simulink model "lookup_nD_TestGen39"  (R2017b)
settings: Solver=FixedStepDiscrete  StartTime=0.0  StopTime=10.0  RelTol=1e-3
model workspace (MAT data in the model file):
  LUTObjLKnD39 = Simulink.LookupTable
  LUTObjLKnD39.Table = Simulink.lookuptable.Table
  LUTObjLKnD39.Table.Value = [4 16 10 4 16 10 4 16 10 4 16 10 ... (2160 elements, 2x5x3x2x3x4x3)]
  LUTObjLKnD39.Table.Dimensions = [2 5 3 2 3 4 3]
  LUTObjLKnD39.Table.DataType = 'double'
  LUTObjLKnD39.Table.FieldName = 'Table'
  LUTObjLKnD39.Breakpoints(1) = Simulink.lookuptable.Breakpoint
  LUTObjLKnD39.Breakpoints(1).Value = [61.721962121; 104.300096243]
  LUTObjLKnD39.Breakpoints(1).TunableSizeName = 'N1'
  LUTObjLKnD39.Breakpoints(1).Dimensions = [2 1]
  LUTObjLKnD39.Breakpoints(1).DataType = 'double'
  LUTObjLKnD39.Breakpoints(1).FieldName = 'BP1'
  LUTObjLKnD39.Breakpoints(2) = Simulink.lookuptable.Breakpoint
  LUTObjLKnD39.Breakpoints(2).Value = [37.260919995; 59.6796023238; 63.5646368852; 96.2573922912; 103.388327939]
  LUTObjLKnD39.Breakpoints(2).TunableSizeName = 'N2'
  LUTObjLKnD39.Breakpoints(2).Dimensions = [5 1]
  LUTObjLKnD39.Breakpoints(2).DataType = 'double'
  LUTObjLKnD39.Breakpoints(2).FieldName = 'BP2'
  LUTObjLKnD39.Breakpoints(3) = Simulink.lookuptable.Breakpoint
  LUTObjLKnD39.Breakpoints(3).Value = [0.658816623389; 20.0277443068; 89.2681267122]
  LUTObjLKnD39.Breakpoints(3).TunableSizeName = 'N3'
  LUTObjLKnD39.Breakpoints(3).Dimensions = [3 1]
  LUTObjLKnD39.Breakpoints(3).DataType = 'double'
  LUTObjLKnD39.Breakpoints(3).FieldName = 'BP3'
  LUTObjLKnD39.Breakpoints(4) = Simulink.lookuptable.Breakpoint
  LUTObjLKnD39.Breakpoints(4).Value = [83.69732351; 108.985900351]
  LUTObjLKnD39.Breakpoints(4).TunableSizeName = 'N4'
  LUTObjLKnD39.Breakpoints(4).Dimensions = [2 1]
  LUTObjLKnD39.Breakpoints(4).DataType = 'double'
  LUTObjLKnD39.Breakpoints(4).FieldName = 'BP4'
  LUTObjLKnD39.Breakpoints(5) = Simulink.lookuptable.Breakpoint
  LUTObjLKnD39.Breakpoints(5).Value = [49.9740707452; 87.8847504391; 124.596963914]
  LUTObjLKnD39.Breakpoints(5).TunableSizeName = 'N5'
  LUTObjLKnD39.Breakpoints(5).Dimensions = [3 1]
  LUTObjLKnD39.Breakpoints(5).DataType = 'double'
  LUTObjLKnD39.Breakpoints(5).FieldName = 'BP5'
  LUTObjLKnD39.Breakpoints(6) = Simulink.lookuptable.Breakpoint
  LUTObjLKnD39.Breakpoints(6).Value = [48.2815081027; 65.4568713881; 80.4779937525; 116.657049975]
  LUTObjLKnD39.Breakpoints(6).TunableSizeName = 'N6'
  LUTObjLKnD39.Breakpoints(6).Dimensions = [4 1]
  LUTObjLKnD39.Breakpoints(6).DataType = 'double'
  LUTObjLKnD39.Breakpoints(6).FieldName = 'BP6'
  LUTObjLKnD39.Breakpoints(7) = Simulink.lookuptable.Breakpoint
  LUTObjLKnD39.Breakpoints(7).Value = [10.6803086369; 11.5286513984; 29.404287558]
  LUTObjLKnD39.Breakpoints(7).TunableSizeName = 'N7'
  LUTObjLKnD39.Breakpoints(7).Dimensions = [3 1]
  LUTObjLKnD39.Breakpoints(7).DataType = 'double'
  LUTObjLKnD39.Breakpoints(7).FieldName = 'BP7'
  LUTObjLKnD39.SupportTunableSize = 0
  LUTObjLKnD39.StructTypeInfo = Simulink.lookuptable.StructTypeInfo
  LUTObjLKnD39.StructTypeInfo.Name = 'LUT'
  LUTObjLKnD39.StructTypeInfo.DataScope = 'Auto'
settings Model: Creator=ktrinh  LastModifiedBy=ktrinh
settings DebuggingCC: ParameterOverflowMsg=none

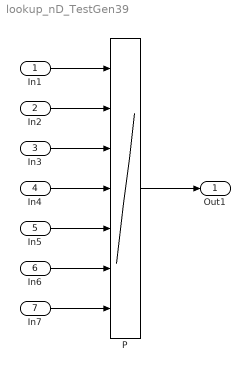
== system lookup_nD_TestGen39 ==
  In1 : Inport  OutMin=0  OutMax=127  PortDimensions=1
  In2 : Inport  Port=2  OutMin=0  OutMax=127
  In3 : Inport  Port=3  OutMin=0  OutMax=127
  In4 : Inport  Port=4  OutMin=0  OutMax=127
  In5 : Inport  Port=5  OutMin=0  OutMax=127
  In6 : Inport  Port=6  OutMin=0  OutMax=127
  In7 : Inport  Port=7  OutMin=0  OutMax=127
  P : Lookup_n-D  NumberOfTableDimensions=7  DataSpecification=Lookup table object  LookupTableObject=LUTObjLKnD39  BreakpointsForDimension3=[5, 7]  Table=reshape(repmat([4 5 6;16 19 20;10 18 23],1,2),[3,3,2])  InterpMethod=Nearest  ExtrapMethod=Clip  UseLastTableValue=on  InternalRulePriority=Speed  OutDataTypeStr=double  RndMeth=Round  SaturateOnIntegerOverflow=on  InputSameDT=on
  Out1 : Outport
  wires:
  In1/1 -> P/1
  In2/1 -> P/2
  In3/1 -> P/3
  In4/1 -> P/4
  In5/1 -> P/5
  In6/1 -> P/6
  In7/1 -> P/7
  P/1 -> Out1/1
